simulink model "QUESTION3_1_CCF"  (R2021a)
settings: Solver=VariableStepAuto  StartTime=0.0  StopTime=10.0  RelTol=1e-3
settings Model: Creator=user  LastModifiedBy=user

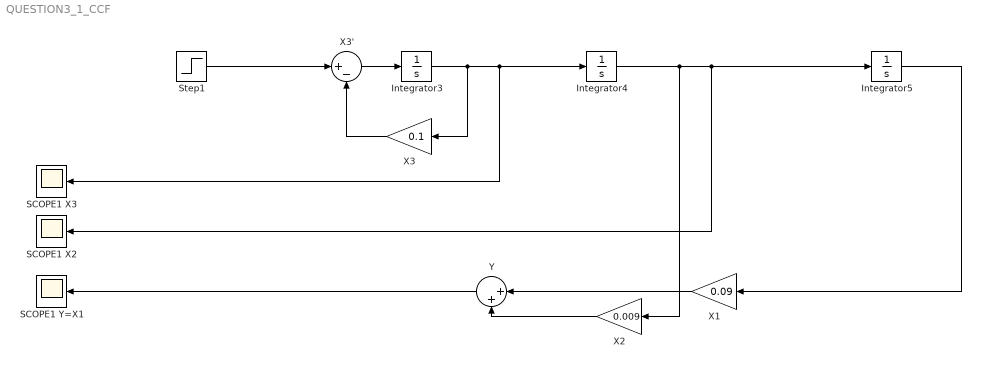
== system QUESTION3_1_CCF ==
  Integrator3 : Integrator
  Integrator4 : Integrator
  Integrator5 : Integrator
  SCOPE1 X2 : Scope
  SCOPE1 X3 : Scope
  SCOPE1 Y=X1 : Scope
  Step1 : Step  SampleTime=0
  X1 : Gain  Gain=0.09
  X2 : Gain  Gain=0.009
  X3 : Gain  Gain=0.1
  X3' : Sum  Inputs=|+-
  Y : Sum  Inputs=|++
  wires:
  X3'/1 -> Integrator3/1
  Integrator3/1 -> SCOPE1 X3/1, Integrator4/1, X3/1
  Integrator4/1 -> Integrator5/1, SCOPE1 X2/1, X2/1
  Step1/1 -> X3'/1
  X3/1 -> X3'/2
  Integrator5/1 -> X1/1
  X2/1 -> Y/2
  X1/1 -> Y/1
  Y/1 -> SCOPE1 Y=X1/1
